simulink library "lib_cal_CAN_msgCount"  (R2020a)
settings: Solver=VariableStepAuto  StartTime=0.0  StopTime=10.0  RelTol=1e-3
settings Model: Creator=zulong.dong  LastModifiedBy=zulong.dong

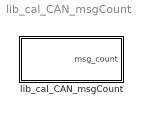
== system lib_cal_CAN_msgCount ==
  lib_cal_CAN_msgCount : Subsystem

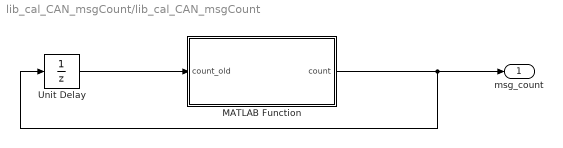
== system lib_cal_CAN_msgCount/lib_cal_CAN_msgCount ==
  MATLAB Function : MATLAB Function  TreatAsAtomicUnit=on
  Unit Delay : UnitDelay  SampleTime=-1  HasFrameUpgradeWarning=on
  msg_count : Outport
  wires:
  MATLAB Function/1(count) -> Unit Delay/1, msg_count/1
  Unit Delay/1 -> MATLAB Function/1(count_old)

== matlab function lib_cal_CAN_msgCount/MATLAB Function ==
  data: count_old input uint8; count output uint8
function count = fcn(count_old)

count = count_old +1;

if count > 15 
    count = uint8(0);
end
